simulink model "model_observer_controller_noise"  (R2024a)
settings: Solver=FixedStepAuto  StartTime=0.0  StopTime=10.0  FixedStep=0.0001  RelTol=1e-3
undefined symbols (not defined in the file or in its folder): A, ampl, B, Bw, C, Cz, D, Dw, Dz, K, L, phi, w
settings Model: Creator=anton  LastModifiedBy=anton

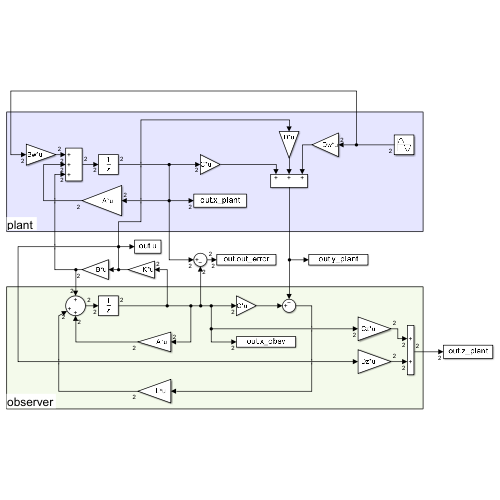
[thumbnail: Simulink's stored preview of the top-level diagram]
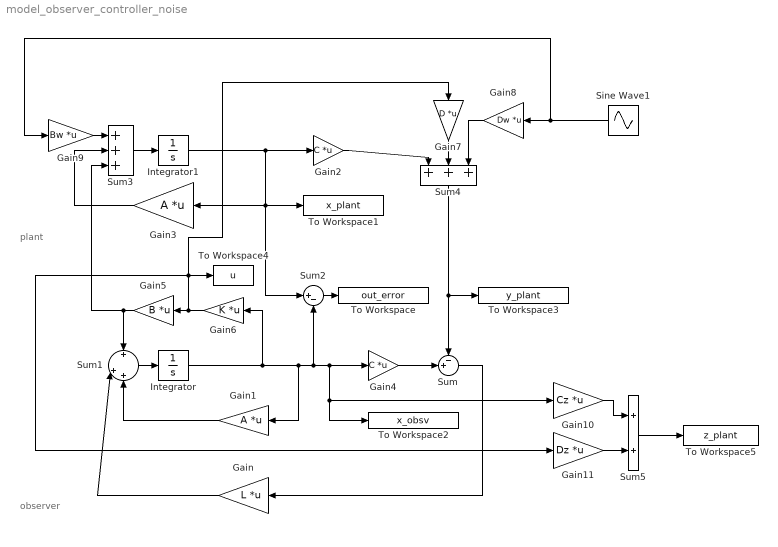
== system model_observer_controller_noise ==
  note: plant
  note: observer
  Gain : Gain  Gain=L  Multiplication=Matrix(K*u)
  Gain1 : Gain  Gain=A  Multiplication=Matrix(K*u)
  Gain10 : Gain  Gain=Cz  Multiplication=Matrix(K*u)
  Gain11 : Gain  Gain=Dz  Multiplication=Matrix(K*u)
  Gain2 : Gain  Gain=C  Multiplication=Matrix(K*u)
  Gain3 : Gain  Gain=A  Multiplication=Matrix(K*u)
  Gain4 : Gain  Gain=C  Multiplication=Matrix(K*u)
  Gain5 : Gain  Gain=B  Multiplication=Matrix(K*u)
  Gain6 : Gain  Gain=K  Multiplication=Matrix(K*u)
  Gain7 : Gain  Gain=D  Multiplication=Matrix(K*u)
  Gain8 : Gain  Gain=Dw  Multiplication=Matrix(K*u)
  Gain9 : Gain  Gain=Bw  Multiplication=Matrix(K*u)
  Integrator : Integrator
  Integrator1 : Integrator
  Sine Wave1 : Sin  Amplitude=ampl  Frequency=w  Phase=phi  SampleTime=0
  Sum : Sum  Inputs=-+|
  Sum1 : Sum  Inputs=+|++
  Sum2 : Sum  Inputs=|+-
  Sum3 : Sum  Inputs=+++
  Sum4 : Sum  Inputs=+++
  Sum5 : Sum
  To Workspace : ToWorkspace  VariableName=out_error  SaveFormat=Timeseries  SampleTime=-1
  To Workspace1 : ToWorkspace  VariableName=x_plant  SaveFormat=Timeseries  SampleTime=-1
  To Workspace2 : ToWorkspace  VariableName=x_obsv  SaveFormat=Timeseries  SampleTime=-1
  To Workspace3 : ToWorkspace  VariableName=y_plant  SaveFormat=Timeseries  SampleTime=-1
  To Workspace4 : ToWorkspace  VariableName=u  SaveFormat=Timeseries  SampleTime=-1
  To Workspace5 : ToWorkspace  VariableName=z_plant  SaveFormat=Timeseries  SampleTime=-1
  wires:
  Gain5/1 -> Sum3/3, Sum1/1
  Gain4/1 -> Sum/2
  Sum3/1 -> Integrator1/1
  Sum2/1 -> To Workspace/1
  Sum1/1 -> Integrator/1
  Integrator/1 -> Gain6/1, Gain1/1, Sum2/2, To Workspace2/1, Gain10/1, Gain4/1
  Sum/1 -> Gain/1
  Integrator1/1 -> Sum2/1, To Workspace1/1, Gain3/1, Gain2/1
  Gain/1 -> Sum1/2
  Gain1/1 -> Sum1/3
  Gain6/1 -> Gain7/1, To Workspace4/1, Gain11/1, Gain5/1
  Gain7/1 -> Sum4/2
  Gain2/1 -> Sum4/1
  Sum4/1 -> Sum/1, To Workspace3/1
  Gain3/1 -> Sum3/2
  Gain8/1 -> Sum4/3
  Gain9/1 -> Sum3/1
  Gain10/1 -> Sum5/1
  Gain11/1 -> Sum5/2
  Sum5/1 -> To Workspace5/1
  Sine Wave1/1 -> Gain8/1, Gain9/1
